simulink model "Fibonacci_out"  (R2014a)
settings: Solver=FixedStepDiscrete  StartTime=0.0  StopTime=50  FixedStep=1  RelTol=1e-3
settings Model: BufferReuse=off  Creator=pdsl  LastModifiedBy=yoshi12
settings DataIOCC: SignalLoggingSaveFormat=ModelDataLogs
settings OptimizationCC: BlockReduction=off  OptimizeBlockIOStorage=off  BufferReuse=off  GlobalBufferReuse=off  ExpressionFolding=off  LocalBlockOutputs=off  OptimizeModelRefInitCode=on  LifeSpan=1
settings DebuggingCC: MultiTaskDSMMsg=warning  MultiTaskCondExecSysMsg=none  StrictBusMsg=ErrorOnBusTreatedAsVector
settings RTWCC: SystemTargetFile=ert.tlc  GenCodeOnly=on  TemplateMakefile=ert_default_tmf  Description=Embedded Coder  GenerateReport=on  ProcessScript=ert_make_rtw_hook  IncludeHyperlinkInReport=on  LaunchReport=on  IncludeERTFirstTime=on  GenerateTraceInfo=on  GenerateTraceReport=on  GenerateTraceReportSl=on  GenerateTraceReportSf=on  GenerateTraceReportEml=on
settings CodeAppCC: IgnoreCustomStorageClasses=off
settings ERTTargetCC: ParMdlRefBuildCompliant=on  CompOptLevelCompliant=on  ConcurrentExecutionCompliant=on  ERTFirstTimeCompliant=on  ModelStepFunctionPrototypeControlCompliant=on  CPPClassGenCompliant=on  InlinedParameterPlacement=Hierarchical  ERTCustomFileTemplate=example_file_process.tlc

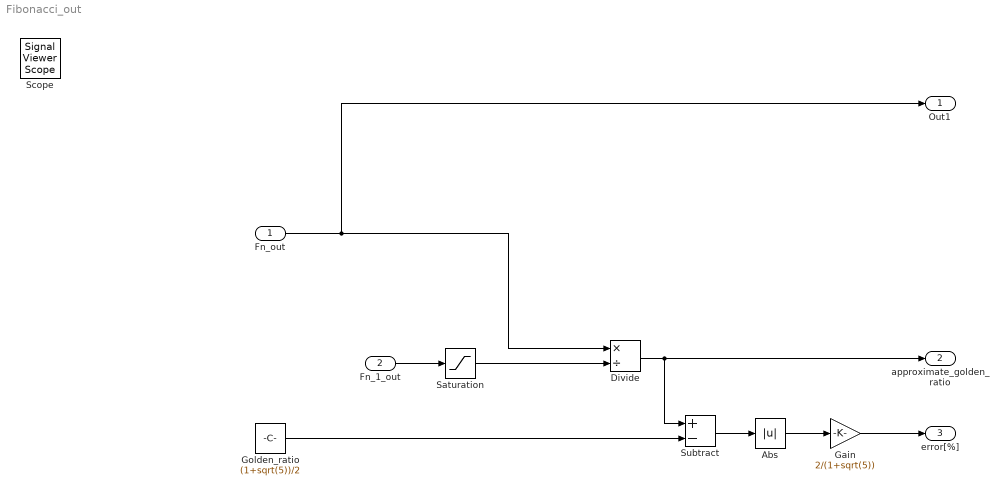
== system Fibonacci_out ==
  Fn_out : Inport
  Fn_1_out : Inport  Port=2
  Abs : Abs
  Divide : Product  Inputs=*/
  Gain : Gain  Gain=2/(1+sqrt(5))
  Golden_ratio : Constant  Value=(1+sqrt(5))/2
  Saturation : Saturate  UpperLimit=inf  LowerLimit=1
  Subtract : Sum  Inputs=+-
  Out1 : Outport
  approximate_golden_ratio : Outport  Port=2
  error[%] : Outport  Port=3
  Scope : SignalViewerScope  IOType=viewer  NumInputPorts=2  ZoomMode=yonly  RefreshTime=0.035000
      settings: YMin=-5~-5  YMax=5~5
  wires:
  Fn_1_out/1 -> Saturation/1
  Saturation/1 -> Divide/2
  Divide/1 -> Subtract/1, approximate_golden_ratio/1
  Golden_ratio/1 -> Subtract/2
  Subtract/1 -> Abs/1
  Gain/1 -> error[%]/1
  Fn_out/1 -> Out1/1, Divide/1
  Abs/1 -> Gain/1
